simulink library "aerolibgravity2"  (Simulink 6.0)
settings: Solver=ode45  SolverMode=SingleTasking  StartTime=0.0  StopTime=10.0  RelTol=1e-3
values from neighbouring files (symbols this model uses):
  s = aeroliblist    [asbhelp.m]
undefined symbols (not defined in the file or in its folder): aeroassertmsg, c, cd, epoch, fm, fn, k, m, maxdef, snorm
libraries: simulink x9, aerolibconvert x8, aerolibutil x2
(part 1 of 2)
settings Model: Creator=sgage  LastModifiedBy=sgage  ExtModeAutoUpdateStatusClock=off  ProdHWDeviceType=Specified
settings DataIOCC: SignalLoggingName=logsOut
settings OptimizationCC: BooleanDataType=off
settings DebuggingCC: CheckExecutionContextPreStartOutputMsg=on  CheckExecutionContextRuntimeOutputMsg=on  SolverPrmCheckMsg=none
settings HardwareCC: ProdHWDeviceType=Specified  TargetUnknown=on
settings GRTTargetCC: LifeSpan=inf
settings SFSimCC: SFSimApplyToAllLibs=on  SFSimBuildMode=Incremental

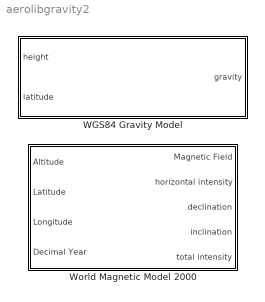
== system aerolibgravity2 ==
  WGS84 Gravity Model : Subsystem  PropExecContextAcrossSSBoundary=on  mask(WGS84 Gravity Model){model=WGS84 Taylor Series, units=Metric (MKS), no_atmos=on, precessing=on, month=February, day=1, year=2000, no_centrifugal=on, action=Warning}
      mask prompts: model "Type of gravity model:"; no_atmos "Exclude Earth's atmosphere"; precessing "Precessing reference frame"; no_centrifugal "No centrifugal effects"; action "Action for out of range input:"
      mask help:
      | Calculate Earth's gravity at a specific location using World Geodetic System (WGS 84).
      |
      | The WGS 84 model is defined as a geocentric equipotential ellipsoid. This model can be found in NIMA TR8350.2,  "Department of Defense World Geodetic System 1984, Its Definition and Relationship with Local Geodetic Systems."
      |
      | Height is entered in the same unit system as selected for gravity. Latitude and longitude (if required) are entered in degrees.
      mask init:
      | [str,ports] = aeroicon('aeroblkgravity','icon');
      mask Help: web(asbhelp);
      mask StyleString: popup(WGS84 Taylor Series|WGS84 Close Approximation|WGS84 Exact),popup(Metric (MKS)|English),checkbox,checkbox,popup(January|February|March|April|May|June|July|August|September|October|November|December),edit,edit,checkbox,popup(None|Warning|Error)
      mask CallbackString: aeroicon('aeroblkgravity')|||aeroicon('aeroblkgravity')|aeroicon('aeroblkgravity')|aeroicon('aeroblkgravity')|aeroicon('aeroblkgravity')||
      mask Display:
      | disp(str);
      | port_label(ports(1).type,ports(1).port,ports(1).txt,'texmode','on');
      | port_label(ports(2).type,ports(2).port,ports(2).txt,'texmode','on');
      | port_label(ports(3).type,ports(3).port,ports(3).txt,'texmode','on');
      | port_label(ports(4).type,ports(4).port,ports(4).txt,'texmode','on');
  World Magnetic Model 2000 : Subsystem  PropExecContextAcrossSSBoundary=on  mask(World Magnetic Model 2000){units=Metric (MKS), time_in=on, month=January, day=1, year=2000, action=Error, h_out=on, dec_out=on, inc_out=on, ti_out=on}
      mask prompts: time_in "Input decimal year"; action "Action for out of range input:"; h_out "Output horizontal intensity"; dec_out "Output declination"; inc_out "Output inclination"; ti_out "Output total intensity"
      mask help:
      | Calculate the Earth's magnetic field at a specific location and time using the World Magnetic Model (WMM). This model is valid for the year 2000 through the year 2005.
      |
      | The WMM-2000 can be found on the web at http://wmm.ngdc.noaa.gov/DoDWMM.shtml and in "British Geological Survey, Technical Report WM/00/17R, Geomagnetism Series".
      |
      | Height is entered in length units of selected unit system. Latitude and longitude are entered in degrees.
      mask init:
      | [ports,dyear,maxdef,epoch,c,cd,fn,fm,snorm,k]=aeroicon('aeroblkwmm','icon');
      mask Help: web(asbhelp);
      mask StyleString: popup(Metric (MKS)|English),checkbox,popup(January|February|March|April|May|June|July|August|September|October|November|December),popup(1|2|3|4|5|6|7|8|9|10|11|12|13|14|15|16|17|18|19|20|21|22|23|24|25|26|27|28|29|30|31),popup(2000|2001|2002|2003|2004|2005),popup(None|Warning|Error),checkbox,checkbox,checkbox,checkbox
      mask CallbackString: |aeroicon('aeroblkwmm');|aeroicon('aeroblkwmm');|aeroicon('aeroblkwmm');|aeroicon('aeroblkwmm');|||||
      mask Display:
      | port_label(ports(1).type,ports(1).port,ports(1).txt);
      | port_label(ports(2).type,ports(2).port,ports(2).txt);
      | port_label(ports(3).type,ports(3).port,ports(3).txt);
      | port_label(ports(4).type,ports(4).port,ports(4).txt);
      | port_label(ports(5).type,ports(5).port,ports(5).txt);
      | port_label(ports(6).type,ports(6).port,ports(6).txt);
      | port_label(ports(7).type,ports(7).port,ports(7).txt);
      | port_label(ports(8).type,ports(8).port,ports(8).txt);
      | port_label(ports(9).type,ports(9).port,ports(9).txt);

== system aerolibgravity2/WGS84 Gravity Model ==
  height : Inport  LatchInput=off
  latitude : Inport  Port=2  LatchInput=off
  Acceleration Conversion : aerolibconvert/Acceleration Conversion  IU=m/s^2  OU=m/s^2
  Angle Conversion : aerolibconvert/Angle Conversion  IU=deg  OU=rad
  Angle Conversion1 : aerolibconvert/Angle Conversion  IU=deg  OU=rad
  Length Conversion : aerolibconvert/Length Conversion  IU=m  OU=m
  WGS84 Gravity S-Function : S-Function  FunctionName=saerogravity2  Parameters=model,units,no_atmos,precessing,month,day,year,no_centrifugal,action  SFunctionModules=aerogravitywgs84
  longitude : Ground
  gravity : Outport
  wires:
  WGS84 Gravity S-Function/1 -> Acceleration Conversion/1
  height/1 -> Length Conversion/1
  latitude/1 -> Angle Conversion1/1
  Length Conversion/1 -> WGS84 Gravity S-Function/1
  Acceleration Conversion/1 -> gravity/1
  Angle Conversion1/1 -> WGS84 Gravity S-Function/2
  longitude/1 -> Angle Conversion/1
  Angle Conversion/1 -> WGS84 Gravity S-Function/3

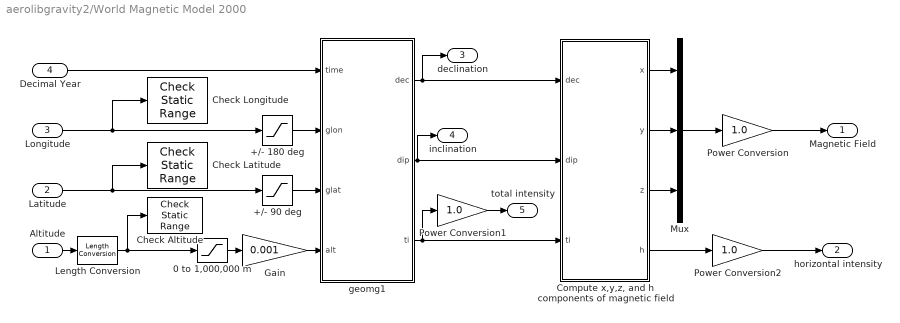
== system aerolibgravity2/World Magnetic Model 2000 ==
  Altitude : Inport  LatchInput=off
  Latitude : Inport  Port=2  LatchInput=off
  Longitude : Inport  Port=3  LatchInput=off
  Decimal Year : Inport  Port=4  LatchInput=off
  +/- 180 deg : Saturate  UpperLimit=180.0  LowerLimit=-180.0
  +/- 90 deg : Saturate  UpperLimit=90.0  LowerLimit=-90.0
  0 to 1,000,000 m : Saturate  UpperLimit=1000000.0  LowerLimit=0
  Check Altitude : simulink/Model Verification/Check  Static Range  Description=0 <= u <= 1000000  max=1000000  max_included=on  min=0  min_included=on  enabled=on  callback=aeroassertmsg('aeroblkwmm','alt');  stopWhenAssertionFail=on  export=off  icon=graphic
  Check Latitude : simulink/Model Verification/Check  Static Range  Description=-90 <= u <= 90  max=90  max_included=on  min=-90  min_included=on  enabled=on  callback=aeroassertmsg('aeroblkwmm','lat');  stopWhenAssertionFail=on  export=off  icon=graphic
  Check Longitude : simulink/Model Verification/Check  Static Range  Description=-180 <= u <= 180  max=180  max_included=on  min=-180  min_included=on  enabled=on  callback=aeroassertmsg('aeroblkwmm','lon');  stopWhenAssertionFail=on  export=off  icon=graphic
  "Compute x,y,z, and h components of magnetic field" : Subsystem  PropExecContextAcrossSSBoundary=on
  Gain : Gain  Gain=0.001  SaturateOnIntegerOverflow=on
  Length Conversion : aerolibconvert/Length Conversion  IU=m  OU=m
  Mux : Mux  Inputs=3
  Power Conversion : Gain  Gain=1.0  SaturateOnIntegerOverflow=on
  Power Conversion1 : Gain  Gain=1.0  SaturateOnIntegerOverflow=on
  Power Conversion2 : Gain  Gain=1.0  SaturateOnIntegerOverflow=on
  geomg1 : Subsystem  PropExecContextAcrossSSBoundary=on
  Magnetic Field : Outport
  horizontal intensity : Outport  Port=2
  declination : Outport  Port=3
  inclination : Outport  Port=4
  total intensity : Outport  Port=5
  wires:
  0 to 1,000,000 m/1 -> Gain/1
  +/- 180 deg/1 -> geomg1/2(glon)
  +/- 90 deg/1 -> geomg1/3(glat)
  Power Conversion2/1 -> horizontal intensity/1
  Power Conversion1/1 -> total intensity/1
  Power Conversion/1 -> Magnetic Field/1
  Mux/1 -> Power Conversion/1
  geomg1/1(dec) -> declination/1, "Compute x,y,z, and h components of magnetic field"/1(dec)
  Gain/1 -> geomg1/4(alt)
  Longitude/1 -> Check Longitude/1, +/- 180 deg/1
  Latitude/1 -> Check Latitude/1, +/- 90 deg/1
  geomg1/3(ti) -> Power Conversion1/1, "Compute x,y,z, and h components of magnetic field"/3(ti)
  geomg1/2(dip) -> inclination/1, "Compute x,y,z, and h components of magnetic field"/2(dip)
  Decimal Year/1 -> geomg1/1(time)
  "Compute x,y,z, and h components of magnetic field"/4(h) -> Power Conversion2/1
  "Compute x,y,z, and h components of magnetic field"/3(z) -> Mux/3
  "Compute x,y,z, and h components of magnetic field"/2(y) -> Mux/2
  "Compute x,y,z, and h components of magnetic field"/1(x) -> Mux/1
  Length Conversion/1 -> Check Altitude/1, 0 to 1,000,000 m/1
  Altitude/1 -> Length Conversion/1

== system aerolibgravity2/World Magnetic Model 2000/Compute x,y,z, and h components of magnetic field ==
  dec : Inport  LatchInput=off
  dip : Inport  Port=2  LatchInput=off
  ti : Inport  Port=3  LatchInput=off
  Demux : Demux  Outputs=2
  Demux1 : Demux  Outputs=2
  Mux : Mux  Inputs=2
  SinCos : aerolibutil/SinCos
  h1 : Product  SaturateOnIntegerOverflow=on
  rTd : Gain  Gain=0.017453292  SaturateOnIntegerOverflow=on
  x1 : Product  SaturateOnIntegerOverflow=on
  y1 : Product  SaturateOnIntegerOverflow=on
  z1 : Product  SaturateOnIntegerOverflow=on
  x : Outport
  y : Outport  Port=2
  z : Outport  Port=3
  h : Outport  Port=4
  wires:
  z1/1 -> z/1
  x1/1 -> x/1
  dip/1 -> Mux/2
  y1/1 -> y/1
  dec/1 -> Mux/1
  Demux1/1 -> y1/1
  Demux1/2 -> z1/1
  Demux/1 -> x1/1
  h1/1 -> h/1, x1/2, y1/2
  Demux/2 -> h1/1
  ti/1 -> h1/2, z1/2
  SinCos/2 -> Demux/1
  SinCos/1 -> Demux1/1
  rTd/1 -> SinCos/1
  Mux/1 -> rTd/1

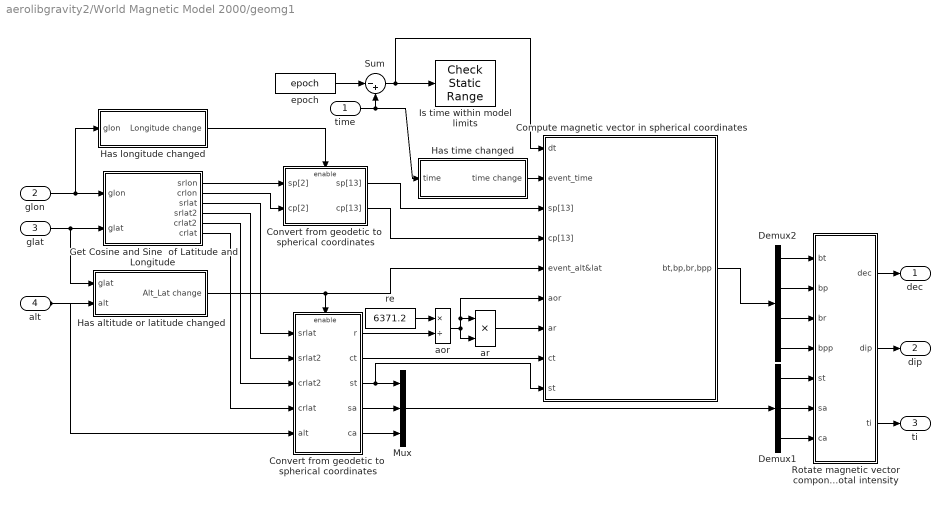
== system aerolibgravity2/World Magnetic Model 2000/geomg1 ==
  time : Inport  LatchInput=off
  glon : Inport  Port=2  LatchInput=off
  glat : Inport  Port=3  LatchInput=off
  alt : Inport  Port=4  LatchInput=off
  Compute magnetic vector in spherical coordinates : Subsystem  TreatAsAtomicUnit=on  PropExecContextAcrossSSBoundary=on
  Convert from geodetic to  spherical coordinates : Subsystem  TreatAsAtomicUnit=on  PropExecContextAcrossSSBoundary=on
  "Convert from geodetic to  spherical coordinates " : Subsystem  PropExecContextAcrossSSBoundary=on
  Demux1 : Demux  Outputs=3
  Demux2 : Demux
  Get Cosine and Sine  of Latitude and Longitude : Subsystem  PropExecContextAcrossSSBoundary=on
  Has altitude or latitude changed : Subsystem  PropExecContextAcrossSSBoundary=on
  "Has longitude changed " : Subsystem  PropExecContextAcrossSSBoundary=on
  Has time changed : Subsystem  AncestorBlock="aerolibatmosratios/WMM 2000/geomg1_/Determine Whether To  Convert Coordinates"  PropExecContextAcrossSSBoundary=on
  Is time within model limits : simulink/Model Verification/Check  Static Range  Description=0 <= u <= 5  max=5  max_included=on  min=0  min_included=on  enabled=on  callback=aeroassertmsg('aeroblkwmm','time');  stopWhenAssertionFail=on  export=off  icon=graphic
  Mux : Mux  Inputs=3
  "Rotate magnetic vector components  to geodetic from spherical and  compute declination, inclination  and total intensity" : Subsystem  PropExecContextAcrossSSBoundary=on
  Sum : Sum  Inputs=|-+  SaturateOnIntegerOverflow=on
  aor : Product  Inputs=*/  SaturateOnIntegerOverflow=on
  ar : Product  SaturateOnIntegerOverflow=on
  epoch : Constant  Value=epoch
  re : Constant  Value=6371.2
  dec : Outport
  dip : Outport  Port=2
  ti : Outport  Port=3
  wires:
  Demux2/3 -> "Rotate magnetic vector components  to geodetic from spherical and  compute declination, inclination  and total intensity"/3(br)
  Demux2/2 -> "Rotate magnetic vector components  to geodetic from spherical and  compute declination, inclination  and total intensity"/2(bp)
  Compute magnetic vector in spherical coordinates/1(bt,bp,br,bpp) -> Demux2/1
  Demux1/3 -> "Rotate magnetic vector components  to geodetic from spherical and  compute declination, inclination  and total intensity"/7(ca)
  Demux1/2 -> "Rotate magnetic vector components  to geodetic from spherical and  compute declination, inclination  and total intensity"/6(sa)
  Demux1/1 -> "Rotate magnetic vector components  to geodetic from spherical and  compute declination, inclination  and total intensity"/5(st)
  Demux2/4 -> "Rotate magnetic vector components  to geodetic from spherical and  compute declination, inclination  and total intensity"/4(bpp)
  Demux2/1 -> "Rotate magnetic vector components  to geodetic from spherical and  compute declination, inclination  and total intensity"/1(bt)
  Mux/1 -> Demux1/1
  Convert from geodetic to  spherical coordinates/5(ca) -> Mux/3
  Convert from geodetic to  spherical coordinates/4(sa) -> Mux/2
  Convert from geodetic to  spherical coordinates/3(st) -> Compute magnetic vector in spherical coordinates/9(st), Mux/1
  epoch/1 -> Sum/1
  Convert from geodetic to  spherical coordinates/2(ct) -> Compute magnetic vector in spherical coordinates/8(ct)
  Get Cosine and Sine  of Latitude and Longitude/6(crlat) -> Convert from geodetic to  spherical coordinates/4(crlat)
  Get Cosine and Sine  of Latitude and Longitude/3(srlat) -> Convert from geodetic to  spherical coordinates/1(srlat)
  "Rotate magnetic vector components  to geodetic from spherical and  compute declination, inclination  and total intensity"/3(ti) -> ti/1
  "Rotate magnetic vector components  to geodetic from spherical and  compute declination, inclination  and total intensity"/2(dip) -> dip/1
  "Rotate magnetic vector components  to geodetic from spherical and  compute declination, inclination  and total intensity"/1(dec) -> dec/1
  ar/1 -> Compute magnetic vector in spherical coordinates/7(ar)
  re/1 -> aor/1
  Convert from geodetic to  spherical coordinates/1(r) -> aor/2
  aor/1 -> ar/1, Compute magnetic vector in spherical coordinates/6(aor), ar/2
  "Convert from geodetic to  spherical coordinates "/2(cp[13]) -> Compute magnetic vector in spherical coordinates/4(cp[13])
  "Convert from geodetic to  spherical coordinates "/1(sp[13]) -> Compute magnetic vector in spherical coordinates/3(sp[13])
  Has altitude or latitude changed/1(Alt_Lat change) -> Compute magnetic vector in spherical coordinates/5(event_alt&lat), Convert from geodetic to  spherical coordinates/Enable
  Get Cosine and Sine  of Latitude and Longitude/5(crlat2) -> Convert from geodetic to  spherical coordinates/3(crlat2)
  Get Cosine and Sine  of Latitude and Longitude/4(srlat2) -> Convert from geodetic to  spherical coordinates/2(srlat2)
  Get Cosine and Sine  of Latitude and Longitude/2(crlon) -> "Convert from geodetic to  spherical coordinates "/2(cp[2])
  Get Cosine and Sine  of Latitude and Longitude/1(srlon) -> "Convert from geodetic to  spherical coordinates "/1(sp[2])
  alt/1 -> Convert from geodetic to  spherical coordinates/5(alt), Has altitude or latitude changed/2(alt)
  glat/1 -> Get Cosine and Sine  of Latitude and Longitude/2(glat), Has altitude or latitude changed/1(glat)
  glon/1 -> Get Cosine and Sine  of Latitude and Longitude/1(glon), "Has longitude changed "/1(glon)
  "Has longitude changed "/1(Longitude change) -> "Convert from geodetic to  spherical coordinates "/Enable
  Has time changed/1(time change) -> Compute magnetic vector in spherical coordinates/2(event_time)
  time/1 -> Sum/2, Has time changed/1(time)
  Sum/1 -> Compute magnetic vector in spherical coordinates/1(dt), Is time within model limits/1

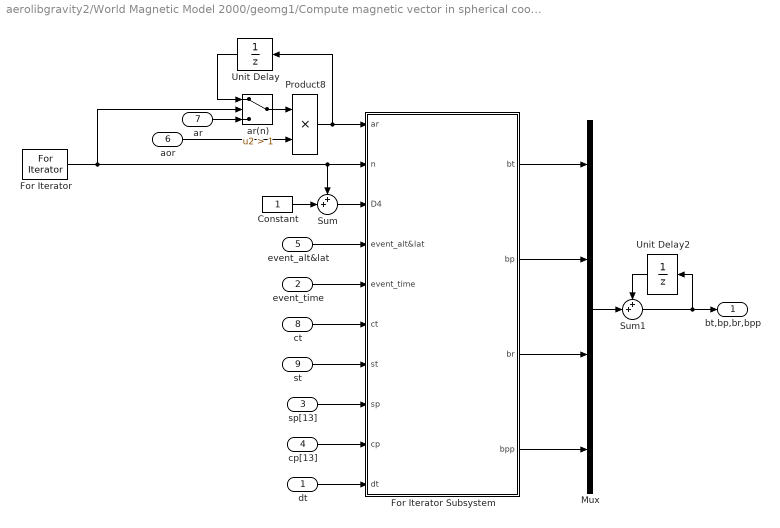
== system aerolibgravity2/World Magnetic Model 2000/geomg1/Compute magnetic vector in spherical coordinates ==
  dt : Inport  LatchInput=off
  event_time : Inport  Port=2  LatchInput=off
  sp[13] : Inport  Port=3  LatchInput=off
  cp[13] : Inport  Port=4  LatchInput=off
  event_alt&lat : Inport  Port=5  LatchInput=off
  aor : Inport  Port=6  LatchInput=off
  ar : Inport  Port=7  LatchInput=off
  ct : Inport  Port=8  LatchInput=off
  st : Inport  Port=9  LatchInput=off
  Constant : Constant
  For Iterator : ForIterator  ResetStates=reset  IterationLimit=maxdef
  For Iterator Subsystem : Subsystem  TreatAsAtomicUnit=on  PropExecContextAcrossSSBoundary=on
  Mux : Mux
  Product8 : Product  SaturateOnIntegerOverflow=on
  Sum : Sum  Inputs=++|  SaturateOnIntegerOverflow=on
  Sum1 : Sum  Inputs=++|  SaturateOnIntegerOverflow=on
  Unit Delay : UnitDelay  Orientation=left  SampleTime=-1
  Unit Delay2 : UnitDelay  Orientation=left  X0=[0 0 0 0]  SampleTime=-1
  ar(n) : Switch  Criteria=u2 > Threshold  Threshold=1  SaturateOnIntegerOverflow=on
  bt,bp,br,bpp : Outport
  wires:
  Sum1/1 -> Unit Delay2/1, bt,bp,br,bpp/1
  Unit Delay2/1 -> Sum1/1
  Mux/1 -> Sum1/2
  For Iterator Subsystem/4(bpp) -> Mux/4
  For Iterator Subsystem/3(br) -> Mux/3
  For Iterator Subsystem/2(bp) -> Mux/2
  For Iterator Subsystem/1(bt) -> Mux/1
  dt/1 -> For Iterator Subsystem/10(dt)
  cp[13]/1 -> For Iterator Subsystem/9(cp)
  sp[13]/1 -> For Iterator Subsystem/8(sp)
  st/1 -> For Iterator Subsystem/7(st)
  ct/1 -> For Iterator Subsystem/6(ct)
  Constant/1 -> Sum/2
  Sum/1 -> For Iterator Subsystem/3(D4)
  ar(n)/1 -> Product8/1
  Product8/1 -> For Iterator Subsystem/1(ar), Unit Delay/1
  Unit Delay/1 -> ar(n)/1
  aor/1 -> Product8/2
  event_time/1 -> For Iterator Subsystem/5(event_time)
  ar/1 -> ar(n)/3
  event_alt&lat/1 -> For Iterator Subsystem/4(event_alt&lat)
  For Iterator/1 -> Sum/1, For Iterator Subsystem/2(n), ar(n)/2

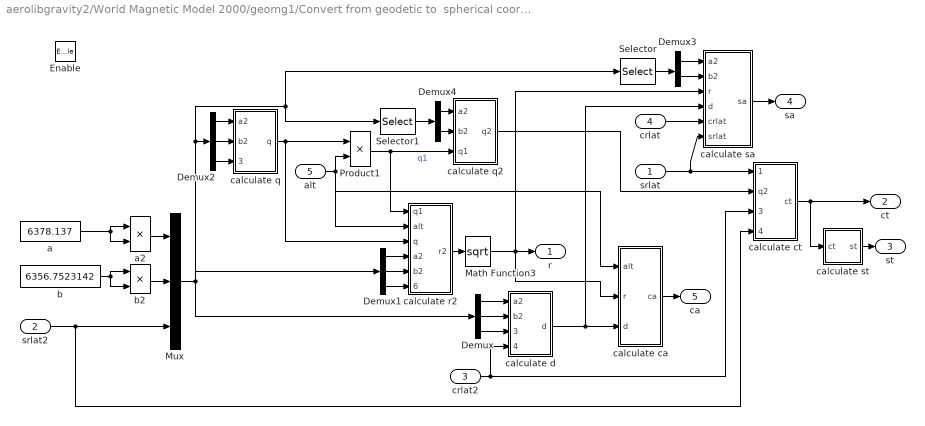
== system aerolibgravity2/World Magnetic Model 2000/geomg1/Convert from geodetic to  spherical coordinates ==
  srlat : Inport  LatchInput=off
  srlat2 : Inport  Port=2  LatchInput=off
  crlat2 : Inport  Port=3  LatchInput=off
  crlat : Inport  Port=4  LatchInput=off
  alt : Inport  Port=5  LatchInput=off
  Enable : EnablePort
  Demux : Demux  Outputs=3
  Demux1 : Demux  Outputs=3
  Demux2 : Demux  Outputs=3
  Demux3 : Demux  Outputs=2
  Demux4 : Demux  Outputs=2
  Math Function3 : Math  Operator=sqrt  SaturateOnIntegerOverflow=on
  Mux : Mux  Inputs=3
  Product1 : Product  SaturateOnIntegerOverflow=on
  Selector : Selector  Elements=[1 2]  InputPortWidth=3
  Selector1 : Selector  Elements=[1 2]  InputPortWidth=3
  a : Constant  Value=6378.137
  a2 : Product  SaturateOnIntegerOverflow=on
  b : Constant  Value=6356.7523142
  b2 : Product  SaturateOnIntegerOverflow=on
  calculate ca : Subsystem  PropExecContextAcrossSSBoundary=on
  calculate ct : Subsystem  PropExecContextAcrossSSBoundary=on
  calculate d : Subsystem  PropExecContextAcrossSSBoundary=on
  calculate q : Subsystem  PropExecContextAcrossSSBoundary=on
  calculate q2 : Subsystem  PropExecContextAcrossSSBoundary=on
  calculate r2 : Subsystem  PropExecContextAcrossSSBoundary=on
  calculate sa : Subsystem  PropExecContextAcrossSSBoundary=on
  calculate st : Subsystem  PropExecContextAcrossSSBoundary=on
  r : Outport
  ct : Outport  Port=2
  st : Outport  Port=3
  sa : Outport  Port=4
  ca : Outport  Port=5
  wires:
  Demux/3 -> calculate d/3(srlat2)
  Demux4/2 -> calculate q2/2(b2)
  Demux4/1 -> calculate q2/1(a2)
  Selector1/1 -> Demux4/1
  Selector/1 -> Demux3/1
  Demux3/2 -> calculate sa/2(b2)
  Demux3/1 -> calculate sa/1(a2)
  Mux/1 -> Selector/1, Selector1/1, Demux2/1, Demux/1, Demux1/1
  Demux2/3 -> calculate q/3(srlat2)
  Demux2/2 -> calculate q/2(b2)
  Demux2/1 -> calculate q/1(a2)
  Demux1/3 -> calculate r2/6(srlat2)
  Demux1/2 -> calculate r2/5(b2)
  Demux1/1 -> calculate r2/4(a2)
  Demux/1 -> calculate d/1(a2)
  Demux/2 -> calculate d/2(b2)
  calculate q2/1(q2) -> calculate ct/2(q2)
  b2/1 -> Mux/2
  b/1 -> b2/1, b2/2
  a2/1 -> Mux/1
  a/1 -> a2/1, a2/2
  calculate sa/1(sa) -> sa/1
  crlat/1 -> calculate sa/5(crlat)
  calculate ca/1(ca) -> ca/1
  calculate d/1(d) -> calculate sa/4(d), calculate ca/3(d)
  Math Function3/1 -> calculate ca/2(r), calculate sa/3(r), r/1
  calculate r2/1(r2) -> Math Function3/1
  calculate st/1(st) -> st/1
  calculate ct/1(ct) -> calculate st/1(ct), ct/1
  srlat/1 -> calculate sa/6(srlat), calculate ct/1(srlat)
  crlat2/1 -> calculate ct/3(crlat2), calculate d/4(crlat2)
  alt/1 -> calculate r2/2(alt), calculate ca/1(alt), Product1/2
  Product1/1 -> calculate r2/1(q1), calculate q2/3(q1)  "q1"
  calculate q/1(q) -> calculate r2/3(q), Product1/1
  srlat2/1 -> Mux/3, calculate ct/4(srlat2)

== system aerolibgravity2/World Magnetic Model 2000/geomg1/Convert from geodetic to  spherical coordinates  ==
  sp[2] : Inport  LatchInput=off
  cp[2] : Inport  Port=2  LatchInput=off
  Enable : EnablePort
  For Iterator Subsystem : Subsystem  AncestorBlock=aerolibatmosratios/WMM 2000/geomg1_/For Iterator Subsystem  TreatAsAtomicUnit=on  PropExecContextAcrossSSBoundary=on
  Mux : Mux  Inputs=3
  Mux1 : Mux  Inputs=3
  cp[1] : Constant
  sp[1] : Constant  Value=0
  sp[13] : Outport  InitialOutput=[ zeros(1,13) ]
  cp[13] : Outport  Port=2  InitialOutput=[ zeros(1,13) ]
  wires:
  sp[1]/1 -> Mux1/1
  cp[1]/1 -> Mux/1
  Mux/1 -> cp[13]/1
  For Iterator Subsystem/2(cp[11]) -> Mux/3
  For Iterator Subsystem/1(sp[11]) -> Mux1/3
  cp[2]/1 -> For Iterator Subsystem/2(cp[2]), Mux/2
  sp[2]/1 -> For Iterator Subsystem/1(sp[2]), Mux1/2
  Mux1/1 -> sp[13]/1

== system aerolibgravity2/World Magnetic Model 2000/geomg1/Get Cosine and Sine  of Latitude and Longitude ==
  glon : Inport  LatchInput=off
  glat : Inport  Port=2  LatchInput=off
  Angle Conversion : aerolibconvert/Angle Conversion  IU=deg  OU=rad
  Demux : Demux  Outputs=2
  Demux1 : Demux  Outputs=2
  Mux : Mux  Inputs=2
  Product : Product  SaturateOnIntegerOverflow=on
  Product1 : Product  SaturateOnIntegerOverflow=on
  SinCos : aerolibutil/SinCos
  srlon : Outport
  crlon : Outport  Port=2
  srlat : Outport  Port=3
  srlat2 : Outport  Port=4
  crlat2 : Outport  Port=5
  crlat : Outport  Port=6
  wires:
  Demux1/2 -> Product1/2, Product1/1, crlat/1
  Demux/2 -> Product/2, Product/1, srlat/1
  Product1/1 -> crlat2/1
  Product/1 -> srlat2/1
  Demux1/1 -> crlon/1
  Demux/1 -> srlon/1
  glat/1 -> Mux/2
  glon/1 -> Mux/1
  SinCos/2 -> Demux1/1
  SinCos/1 -> Demux/1
  Mux/1 -> Angle Conversion/1
  Angle Conversion/1 -> SinCos/1

== system aerolibgravity2/World Magnetic Model 2000/geomg1/Has altitude or latitude changed ==
  glat : Inport  LatchInput=off
  alt : Inport  Port=2  LatchInput=off
  Logical Operator : Logic  Operator=OR  AllPortsSameDT=off
  Relational Operator : RelationalOperator  Operator=~=
  Relational Operator1 : RelationalOperator  Operator=~=
  oalt : Memory  X0=-1000
  olat : Memory  X0=-1000
  Alt_Lat change : Outport
  wires:
  Logical Operator/1 -> Alt_Lat change/1
  glat/1 -> olat/1, Relational Operator/1
  Relational Operator1/1 -> Logical Operator/2
  Relational Operator/1 -> Logical Operator/1
  oalt/1 -> Relational Operator1/2
  olat/1 -> Relational Operator/2
  alt/1 -> oalt/1, Relational Operator1/1

== system aerolibgravity2/World Magnetic Model 2000/geomg1/Has longitude changed  ==
  glon : Inport  LatchInput=off
  Relational Operator : RelationalOperator  Operator=~=
  olon : Memory  X0=-1000
  Longitude change : Outport
  wires:
  Relational Operator/1 -> Longitude change/1
  glon/1 -> olon/1, Relational Operator/1
  olon/1 -> Relational Operator/2

== system aerolibgravity2/World Magnetic Model 2000/geomg1/Has time changed ==
  time : Inport  LatchInput=off
  Relational Operator : RelationalOperator  Operator=~=
  otime : Memory  X0=-1000
  time change : Outport
  wires:
  otime/1 -> Relational Operator/2
  time/1 -> Relational Operator/1, otime/1
  Relational Operator/1 -> time change/1

== system aerolibgravity2/World Magnetic Model 2000/geomg1/Rotate magnetic vector components  to geodetic from spherical and  compute declination, inclination  and total intensity ==
  bt : Inport  LatchInput=off
  bp : Inport  Port=2  LatchInput=off
  br : Inport  Port=3  LatchInput=off
  bpp : Inport  Port=4  LatchInput=off
  st : Inport  Port=5  LatchInput=off
  sa : Inport  Port=6  LatchInput=off
  ca : Inport  Port=7  LatchInput=off
  Calculate bx : Subsystem  PropExecContextAcrossSSBoundary=on
  Calculate by : Subsystem  PropExecContextAcrossSSBoundary=on
  Calculate bz : Subsystem  AncestorBlock=aerolibatmosratios/WMM 2000/geomg1_/Subsystem1/Calculate bx  PropExecContextAcrossSSBoundary=on
  "Compute declination, inclination,  and total intensity" : Subsystem  PropExecContextAcrossSSBoundary=on
  Demux : Demux
  Demux1 : Demux
  Mux : Mux
  dec : Outport
  dip : Outport  Port=2
  ti : Outport  Port=3
  wires:
  "Compute declination, inclination,  and total intensity"/2(dip) -> dip/1
  "Compute declination, inclination,  and total intensity"/1(dec) -> dec/1
  Calculate bz/1(bz) -> "Compute declination, inclination,  and total intensity"/3(bz)
  Calculate bx/1(bx) -> "Compute declination, inclination,  and total intensity"/2(bx)
  Calculate by/1(by) -> "Compute declination, inclination,  and total intensity"/1(by)
  "Compute declination, inclination,  and total intensity"/3(ti) -> ti/1
  Demux1/4 -> Calculate bz/4(br)
  Demux1/3 -> Calculate bz/3(bt)
  Demux1/2 -> Calculate bz/2(sa)
  Demux1/1 -> Calculate bz/1(ca)
  Mux/1 -> Demux1/1, Demux/1
  Demux/4 -> Calculate bx/4(br)
  Demux/3 -> Calculate bx/3(bt)
  Demux/2 -> Calculate bx/2(sa)
  Demux/1 -> Calculate bx/1(ca)
  br/1 -> Mux/4
  bt/1 -> Mux/3
  sa/1 -> Mux/2
  ca/1 -> Mux/1
  bp/1 -> Calculate by/1(bp)
  bpp/1 -> Calculate by/3(bpp)
  st/1 -> Calculate by/2(st)

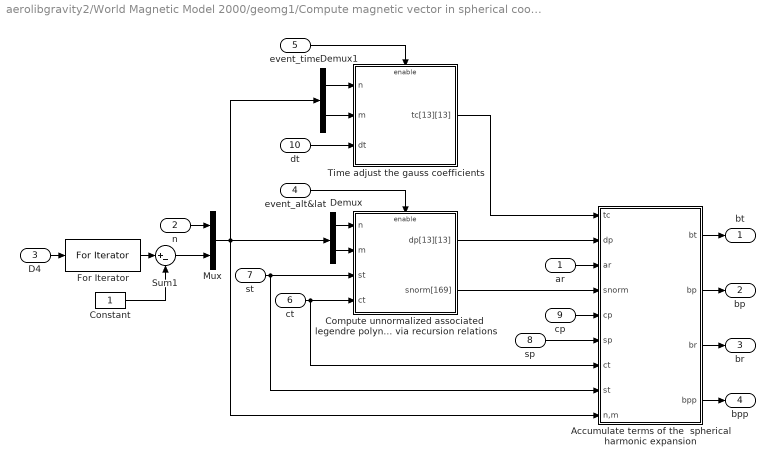
== system aerolibgravity2/World Magnetic Model 2000/geomg1/Compute magnetic vector in spherical coordinates/For Iterator Subsystem ==
  ar : Inport  LatchInput=off
  n : Inport  Port=2  LatchInput=off
  D4 : Inport  Port=3  LatchInput=off
  event_alt&lat : Inport  Port=4  LatchInput=off
  event_time : Inport  Port=5  LatchInput=off
  ct : Inport  Port=6  LatchInput=off
  st : Inport  Port=7  LatchInput=off
  sp : Inport  Port=8  LatchInput=off
  cp : Inport  Port=9  LatchInput=off
  dt : Inport  Port=10  LatchInput=off
  Accumulate terms of the  spherical harmonic expansion : Subsystem  PropExecContextAcrossSSBoundary=on
  Compute unnormalized associated  legendre polynomials and  derivatives via recursion relations : Subsystem  TreatAsAtomicUnit=on  PropExecContextAcrossSSBoundary=on
  Constant : Constant
  Demux : Demux  Outputs=2
  Demux1 : Demux  Outputs=2
  For Iterator : ForIterator  ResetStates=reset  IterationSource=external  IterationLimit=maxdef
  Mux : Mux  Inputs=2
  Sum1 : Sum  Inputs=|+-  SaturateOnIntegerOverflow=on
  Time adjust the gauss coefficients : Subsystem  TreatAsAtomicUnit=on  PropExecContextAcrossSSBoundary=on
  bt : Outport
  bp : Outport  Port=2
  br : Outport  Port=3
  bpp : Outport  Port=4
  wires:
  Accumulate terms of the  spherical harmonic expansion/4(bpp) -> bpp/1
  Sum1/1 -> Mux/2
  For Iterator/1 -> Sum1/1
  Demux1/2 -> Time adjust the gauss coefficients/2(m)
  Demux1/1 -> Time adjust the gauss coefficients/1(n)
  Demux/2 -> Compute unnormalized associated  legendre polynomials and  derivatives via recursion relations/2(m)
  Demux/1 -> Compute unnormalized associated  legendre polynomials and  derivatives via recursion relations/1(n)
  n/1 -> Mux/1
  Mux/1 -> Accumulate terms of the  spherical harmonic expansion/9(n,m), Demux1/1, Demux/1
  Time adjust the gauss coefficients/1(tc[13][13]) -> Accumulate terms of the  spherical harmonic expansion/1(tc)
  ar/1 -> Accumulate terms of the  spherical harmonic expansion/3(ar)
  Accumulate terms of the  spherical harmonic expansion/2(bp) -> bp/1
  Accumulate terms of the  spherical harmonic expansion/1(bt) -> bt/1
  Accumulate terms of the  spherical harmonic expansion/3(br) -> br/1
  Compute unnormalized associated  legendre polynomials and  derivatives via recursion relations/1(dp[13][13]) -> Accumulate terms of the  spherical harmonic expansion/2(dp)
  Compute unnormalized associated  legendre polynomials and  derivatives via recursion relations/2(snorm[169]) -> Accumulate terms of the  spherical harmonic expansion/4(snorm)
  sp/1 -> Accumulate terms of the  spherical harmonic expansion/6(sp)
  cp/1 -> Accumulate terms of the  spherical harmonic expansion/5(cp)
  ct/1 -> Accumulate terms of the  spherical harmonic expansion/7(ct), Compute unnormalized associated  legendre polynomials and  derivatives via recursion relations/4(ct)
  st/1 -> Accumulate terms of the  spherical harmonic expansion/8(st), Compute unnormalized associated  legendre polynomials and  derivatives via recursion relations/3(st)
  dt/1 -> Time adjust the gauss coefficients/3(dt)
  event_time/1 -> Time adjust the gauss coefficients/Enable
  Constant/1 -> Sum1/2
  event_alt&lat/1 -> Compute unnormalized associated  legendre polynomials and  derivatives via recursion relations/Enable
  D4/1 -> For Iterator/1

== system aerolibgravity2/World Magnetic Model 2000/geomg1/Convert from geodetic to  spherical coordinates/calculate ca ==
  alt : Inport  LatchInput=off
  r : Inport  Port=2  LatchInput=off
  d : Inport  Port=3  LatchInput=off
  Product11 : Product  Inputs=/*  SaturateOnIntegerOverflow=on
  Sum8 : Sum  Inputs=|++  SaturateOnIntegerOverflow=on
  ca : Outport
  wires:
  Product11/1 -> ca/1
  d/1 -> Sum8/2
  alt/1 -> Sum8/1
  r/1 -> Product11/1
  Sum8/1 -> Product11/2

== system aerolibgravity2/World Magnetic Model 2000/geomg1/Convert from geodetic to  spherical coordinates/calculate ct ==
  srlat : Inport  LatchInput=off
  q2 : Inport  Port=2  LatchInput=off
  crlat2 : Inport  Port=3  LatchInput=off
  srlat2 : Inport  Port=4  LatchInput=off
  Math Function1 : Math  Operator=sqrt  SaturateOnIntegerOverflow=on
  Product3 : Product  SaturateOnIntegerOverflow=on
  Product4 : Product  Inputs=*/  SaturateOnIntegerOverflow=on
  Sum3 : Sum  Inputs=|++  SaturateOnIntegerOverflow=on
  ct : Outport
  wires:
  Product3/1 -> Sum3/2
  srlat2/1 -> Sum3/1
  q2/1 -> Product3/2
  crlat2/1 -> Product3/1
  Product4/1 -> ct/1
  srlat/1 -> Product4/1
  Math Function1/1 -> Product4/2
  Sum3/1 -> Math Function1/1

== system aerolibgravity2/World Magnetic Model 2000/geomg1/Convert from geodetic to  spherical coordinates/calculate d ==
  a2 : Inport  LatchInput=off
  b2 : Inport  Port=2  LatchInput=off
  srlat2 : Inport  Port=3  LatchInput=off
  crlat2 : Inport  Port=4  LatchInput=off
  Math Function4 : Math  Operator=sqrt  SaturateOnIntegerOverflow=on
  Product10 : Product  SaturateOnIntegerOverflow=on
  Product9 : Product  SaturateOnIntegerOverflow=on
  Sum7 : Sum  Inputs=++|  SaturateOnIntegerOverflow=on
  d : Outport
  wires:
  Math Function4/1 -> d/1  "d"
  srlat2/1 -> Product10/2
  b2/1 -> Product10/1
  a2/1 -> Product9/2
  crlat2/1 -> Product9/1
  Product10/1 -> Sum7/2
  Product9/1 -> Sum7/1
  Sum7/1 -> Math Function4/1

== system aerolibgravity2/World Magnetic Model 2000/geomg1/Convert from geodetic to  spherical coordinates/calculate q ==
  a2 : Inport  LatchInput=off
  b2 : Inport  Port=2  LatchInput=off
  srlat2 : Inport  Port=3  LatchInput=off
  Math Function : Math  Operator=sqrt  SaturateOnIntegerOverflow=on
  Product : Product  SaturateOnIntegerOverflow=on
  Sum : Sum  Inputs=|-+  SaturateOnIntegerOverflow=on
  Sum1 : Sum  Inputs=|-+  SaturateOnIntegerOverflow=on
  q : Outport
  wires:
  b2/1 -> Sum1/1
  Math Function/1 -> q/1  "q"
  a2/1 -> Sum1/2, Sum/2
  Sum1/1 -> Product/2  "c2"
  srlat2/1 -> Product/1
  Sum/1 -> Math Function/1
  Product/1 -> Sum/1

== system aerolibgravity2/World Magnetic Model 2000/geomg1/Convert from geodetic to  spherical coordinates/calculate q2 ==
  a2 : Inport  LatchInput=off
  b2 : Inport  Port=2  LatchInput=off
  q1 : Inport  Port=3  LatchInput=off
  Product2 : Product  Inputs=**//  SaturateOnIntegerOverflow=on
  Sum1 : Sum  Inputs=++|  SaturateOnIntegerOverflow=on
  Sum2 : Sum  Inputs=++|  SaturateOnIntegerOverflow=on
  q2 : Outport
  wires:
  Product2/1 -> q2/1  "q2"
  b2/1 -> Sum1/2
  q1/1 -> Sum1/1, Sum2/2
  a2/1 -> Sum2/1
  Sum2/1 -> Product2/2, Product2/1
  Sum1/1 -> Product2/3, Product2/4

== system aerolibgravity2/World Magnetic Model 2000/geomg1/Convert from geodetic to  spherical coordinates/calculate r2 ==
  q1 : Inport  Orientation=down  LatchInput=off
  alt : Inport  Port=2  LatchInput=off
  q : Inport  Port=3  LatchInput=off
  a2 : Inport  Port=4  LatchInput=off
  b2 : Inport  Port=5  LatchInput=off
  srlat2 : Inport  Orientation=up  Port=6  LatchInput=off
  Gain : Gain  Orientation=down  Gain=2  SaturateOnIntegerOverflow=on
  Product6 : Product  SaturateOnIntegerOverflow=on
  Product7 : Product  Inputs=//*  SaturateOnIntegerOverflow=on
  Product8 : Product  Orientation=up  SaturateOnIntegerOverflow=on
  Sum5 : Sum  Inputs=+++  SaturateOnIntegerOverflow=on
  Sum6 : Sum  Inputs=|+-  SaturateOnIntegerOverflow=on
  Sum9 : Sum  Inputs=|+-  SaturateOnIntegerOverflow=on
  a4 : Product  SaturateOnIntegerOverflow=on
  b4 : Product  SaturateOnIntegerOverflow=on
  r2 : Outport
  wires:
  b2/1 -> b4/1, b4/2
  b4/1 -> Sum9/2
  Sum5/1 -> r2/1  "r2"
  srlat2/1 -> Product8/2
  a2/1 -> a4/2, a4/1
  alt/1 -> Product6/1, Product6/2
  q/1 -> Product7/1, Product7/2
  q1/1 -> Gain/1
  a4/1 -> Sum6/1, Sum9/1
  Sum9/1 -> Product8/1  "c4"
  Product8/1 -> Sum6/2
  Sum6/1 -> Product7/3
  Product7/1 -> Sum5/3
  Gain/1 -> Sum5/1
  Product6/1 -> Sum5/2

== system aerolibgravity2/World Magnetic Model 2000/geomg1/Convert from geodetic to  spherical coordinates/calculate sa ==
  a2 : Inport  LatchInput=off
  b2 : Inport  Port=2  LatchInput=off
  r : Inport  Port=3  LatchInput=off
  d : Inport  Port=4  LatchInput=off
  crlat : Inport  Port=5  LatchInput=off
  srlat : Inport  Port=6  LatchInput=off
  Product12 : Product  Inputs=*//**  SaturateOnIntegerOverflow=on
  Sum1 : Sum  Inputs=|-+  SaturateOnIntegerOverflow=on
  sa : Outport
  wires:
  crlat/1 -> Product12/4
  Product12/1 -> sa/1
  a2/1 -> Sum1/2
  b2/1 -> Sum1/1
  srlat/1 -> Product12/5
  d/1 -> Product12/3
  r/1 -> Product12/2
  Sum1/1 -> Product12/1  "c2"

== system aerolibgravity2/World Magnetic Model 2000/geomg1/Convert from geodetic to  spherical coordinates/calculate st ==
  ct : Inport  LatchInput=off
  Constant : Constant
  Math Function2 : Math  Operator=sqrt  SaturateOnIntegerOverflow=on
  Product5 : Product  SaturateOnIntegerOverflow=on
  Sum4 : Sum  Inputs=|-+  SaturateOnIntegerOverflow=on
  st : Outport
  wires:
  Math Function2/1 -> st/1
  ct/1 -> Product5/2, Product5/1
  Constant/1 -> Sum4/2
  Sum4/1 -> Math Function2/1
  Product5/1 -> Sum4/1

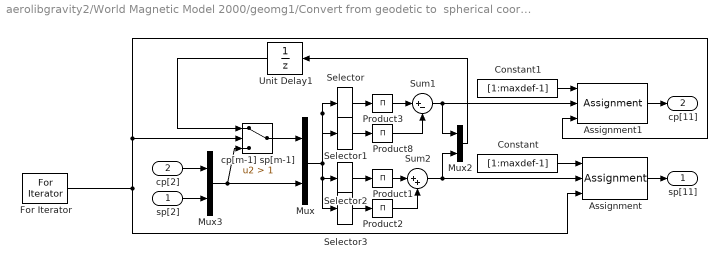
== system aerolibgravity2/World Magnetic Model 2000/geomg1/Convert from geodetic to  spherical coordinates /For Iterator Subsystem ==
  sp[2] : Inport  LatchInput=off
  cp[2] : Inport  Port=2  LatchInput=off
  Assignment : Assignment  ElementSrc=External  DiagnosticForDimensions=Error
  Assignment1 : Assignment  ElementSrc=External  DiagnosticForDimensions=Error
  Constant : Constant  Value=[1:maxdef-1]
  Constant1 : Constant  Value=[1:maxdef-1]
  For Iterator : ForIterator  IterationLimit=maxdef-1  IterationVariableDataType=double
  Mux : Mux  Inputs=[2 2]
  Mux2 : Mux  Inputs=2
  Mux3 : Mux  Inputs=2
  Product{1..3,8} (4 alike) : Product  Inputs=1  SaturateOnIntegerOverflow=on
  Selector : Selector  Elements=[1 3]  InputPortWidth=4
  Selector1 : Selector  Elements=[2 4]  InputPortWidth=4
  Selector2 : Selector  Elements=[1 4]  InputPortWidth=4
  Selector3 : Selector  Elements=[2 3]  InputPortWidth=4
  Sum1 : Sum  Inputs=|+-  SaturateOnIntegerOverflow=on
  Sum2 : Sum  Inputs=|++  SaturateOnIntegerOverflow=on
  Unit Delay1 : UnitDelay  Orientation=left  SampleTime=-1
  cp[m-1] sp[m-1] : Switch  Criteria=u2 > Threshold  Threshold=1  SaturateOnIntegerOverflow=on
  sp[11] : Outport
  cp[11] : Outport  Port=2
  wires:
  Mux3/1 -> cp[m-1] sp[m-1]/3, Mux/2
  Mux2/1 -> Unit Delay1/1
  Selector3/1 -> Product2/1
  Selector2/1 -> Product1/1
  Selector1/1 -> Product8/1
  Mux/1 -> Selector2/1, Selector3/1, Selector1/1, Selector/1
  Selector/1 -> Product3/1
  cp[m-1] sp[m-1]/1 -> Mux/1
  Constant1/1 -> Assignment1/1
  For Iterator/1 -> Assignment/3, cp[m-1] sp[m-1]/2, Assignment1/3
  sp[2]/1 -> Mux3/2
  cp[2]/1 -> Mux3/1
  Assignment1/1 -> cp[11]/1
  Product3/1 -> Sum1/1
  Product8/1 -> Sum1/2
  Product1/1 -> Sum2/1
  Product2/1 -> Sum2/2
  Sum2/1 -> Mux2/2, Assignment/2
  Sum1/1 -> Mux2/1, Assignment1/2
  Unit Delay1/1 -> cp[m-1] sp[m-1]/1
  Assignment/1 -> sp[11]/1
  Constant/1 -> Assignment/1

== system aerolibgravity2/World Magnetic Model 2000/geomg1/Rotate magnetic vector components  to geodetic from spherical and  compute declination, inclination  and total intensity/Calculate bx ==
  ca : Inport  LatchInput=off
  sa : Inport  Port=2  LatchInput=off
  bt : Inport  Port=3  LatchInput=off
  br : Inport  Port=4  LatchInput=off
  Product1 : Product  SaturateOnIntegerOverflow=on
  Product4 : Product  SaturateOnIntegerOverflow=on
  Sum1 : Sum  Inputs=|--  SaturateOnIntegerOverflow=on
  bx : Outport
  wires:
  sa/1 -> Product4/2
  Sum1/1 -> bx/1  "bx"
  ca/1 -> Product1/1
  br/1 -> Product4/1
  bt/1 -> Product1/2
  Product4/1 -> Sum1/2
  Product1/1 -> Sum1/1

== system aerolibgravity2/World Magnetic Model 2000/geomg1/Rotate magnetic vector components  to geodetic from spherical and  compute declination, inclination  and total intensity/Calculate by ==
  bp : Inport  LatchInput=off
  st : Inport  Port=2  LatchInput=off
  bpp : Inport  Port=3  LatchInput=off
  Product : Product  Inputs=*/  SaturateOnIntegerOverflow=on
  Switch : Switch  Criteria=u2 ~= 0  SaturateOnIntegerOverflow=on
  by : Outport
  wires:
  bpp/1 -> Switch/3
  Switch/1 -> by/1  "by"
  bp/1 -> Product/1
  Product/1 -> Switch/1
  st/1 -> Switch/2, Product/2

== system aerolibgravity2/World Magnetic Model 2000/geomg1/Rotate magnetic vector components  to geodetic from spherical and  compute declination, inclination  and total intensity/Calculate bz ==
  ca : Inport  LatchInput=off
  sa : Inport  Port=2  LatchInput=off
  bt : Inport  Port=3  LatchInput=off
  br : Inport  Port=4  LatchInput=off
  Product1 : Product  SaturateOnIntegerOverflow=on
  Product4 : Product  SaturateOnIntegerOverflow=on
  Sum1 : Sum  Inputs=|+-  SaturateOnIntegerOverflow=on
  bz : Outport
  wires:
  Product1/1 -> Sum1/1
  Product4/1 -> Sum1/2
  bt/1 -> Product1/2
  br/1 -> Product4/1
  sa/1 -> Product1/1
  Sum1/1 -> bz/1  "bz"
  ca/1 -> Product4/2

== system aerolibgravity2/World Magnetic Model 2000/geomg1/Rotate magnetic vector components  to geodetic from spherical and  compute declination, inclination  and total intensity/Compute declination, inclination,  and total intensity ==
  by : Inport  LatchInput=off
  bx : Inport  Port=2  LatchInput=off
  bz : Inport  Port=3  LatchInput=off
  Angle Conversion1 : aerolibconvert/Angle Conversion  IU=rad  OU=deg
  Angle Conversion2 : aerolibconvert/Angle Conversion  IU=rad  OU=deg
  Math Function : Math  Operator=sqrt  SaturateOnIntegerOverflow=on
  Math Function1 : Math  Operator=sqrt  SaturateOnIntegerOverflow=on
  Product : Product  SaturateOnIntegerOverflow=on
  Product1 : Product  SaturateOnIntegerOverflow=on
  Product2 : Product  SaturateOnIntegerOverflow=on
  Sum : Sum  Inputs=|++  SaturateOnIntegerOverflow=on
  Sum1 : Sum  Inputs=++|  SaturateOnIntegerOverflow=on
  Trigonometric Function : Trigonometry  Operator=atan2
  Trigonometric Function1 : Trigonometry  Operator=atan2
  dec : Outport
  dip : Outport  Port=2
  ti : Outport  Port=3
  wires:
  Angle Conversion1/1 -> dec/1
  Trigonometric Function1/1 -> Angle Conversion1/1
  Angle Conversion2/1 -> dip/1
  Trigonometric Function/1 -> Angle Conversion2/1
  Math Function1/1 -> Trigonometric Function/2
  Sum1/1 -> Math Function/1
  Product2/1 -> Sum1/1
  Sum/1 -> Sum1/2, Math Function1/1
  Product1/1 -> Sum/2
  Product/1 -> Sum/1
  bz/1 -> Trigonometric Function/1, Product2/2, Product2/1
  bx/1 -> Trigonometric Function1/2, Product1/2, Product1/1
  by/1 -> Trigonometric Function1/1, Product/2, Product/1
  Math Function/1 -> ti/1

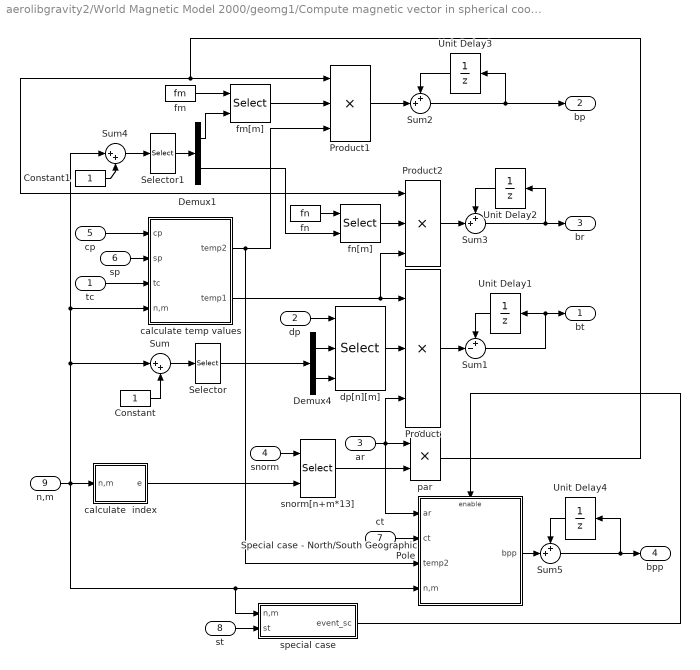
== system aerolibgravity2/World Magnetic Model 2000/geomg1/Compute magnetic vector in spherical coordinates/For Iterator Subsystem/Accumulate terms of the  spherical harmonic expansion ==
  tc : Inport  LatchInput=off
  dp : Inport  Port=2  LatchInput=off
  ar : Inport  Port=3  LatchInput=off
  snorm : Inport  Port=4  LatchInput=off
  cp : Inport  Port=5  LatchInput=off
  sp : Inport  Port=6  LatchInput=off
  ct : Inport  Port=7  LatchInput=off
  st : Inport  Port=8  LatchInput=off
  n,m : Inport  Port=9  LatchInput=off
  Constant : Constant
  Constant1 : Constant
  Demux1 : Demux  Outputs=2
  Demux4 : Demux  Outputs=2
  Product : Product  Inputs=3  SaturateOnIntegerOverflow=on
  Product1 : Product  Inputs=3  SaturateOnIntegerOverflow=on
  Product2 : Product  Inputs=3  SaturateOnIntegerOverflow=on
  Selector : Selector  Elements=[2 1]  InputPortWidth=2
  Selector1 : Selector  Elements=[2 1]  InputPortWidth=2
  Special case - North/South Geographic Pole : Subsystem  TreatAsAtomicUnit=on  PropExecContextAcrossSSBoundary=on
  Sum : Sum  Inputs=|++  SaturateOnIntegerOverflow=on
  Sum1 : Sum  Inputs=+-|  SaturateOnIntegerOverflow=on
  Sum2 : Sum  Inputs=++|  SaturateOnIntegerOverflow=on
  Sum3 : Sum  Inputs=++|  SaturateOnIntegerOverflow=on
  Sum4 : Sum  Inputs=|++  SaturateOnIntegerOverflow=on
  Sum5 : Sum  Inputs=++|  SaturateOnIntegerOverflow=on
  Unit Delay{1..4} (4 alike) : UnitDelay  Orientation=left  SampleTime=-1
  calculate  index : Subsystem  PropExecContextAcrossSSBoundary=on
  calculate temp values : Subsystem  PropExecContextAcrossSSBoundary=on
  dp[n][m] : Selector  InputType=Matrix  ElementSrc=External  Elements=[1 3]  RowSrc=External  ColumnSrc=External  InputPortWidth=maxdef+1
  fm : Constant  Value=fm
  fm[m] : Selector  ElementSrc=External  Elements=[1 3]  InputPortWidth=maxdef+1
  fn : Constant  Value=fn
  fn[m] : Selector  ElementSrc=External  Elements=[1 3]  InputPortWidth=maxdef+1
  par : Product  SaturateOnIntegerOverflow=on
  snorm[n+m*13] : Selector  ElementSrc=External  Elements=[1 3]  InputPortWidth=(maxdef+1)*(maxdef+1)
  special case : Subsystem  PropExecContextAcrossSSBoundary=on
  bt : Outport
  bp : Outport  Port=2
  br : Outport  Port=3
  bpp : Outport  Port=4
  wires:
  special case/1(event_sc) -> Special case - North/South Geographic Pole/Enable
  st/1 -> special case/2(st)
  ct/1 -> Special case - North/South Geographic Pole/2(ct)
  Demux1/2 -> fn[m]/2
  Demux1/1 -> fm[m]/2
  Selector1/1 -> Demux1/1
  Sum4/1 -> Selector1/1
  Constant1/1 -> Sum4/2
  Demux4/2 -> dp[n][m]/3
  Demux4/1 -> dp[n][m]/2
  Selector/1 -> Demux4/1
  Constant/1 -> Sum/2
  Sum/1 -> Selector/1
  tc/1 -> calculate temp values/3(tc)
  Unit Delay2/1 -> Sum3/1
  Sum3/1 -> Unit Delay2/1, br/1
  Product2/1 -> Sum3/2
  fm[m]/1 -> Product1/2
  fn[m]/1 -> Product2/2
  sp/1 -> calculate temp values/2(sp)
  cp/1 -> calculate temp values/1(cp)
  n,m/1 -> special case/1(n,m), Special case - North/South Geographic Pole/4(n,m), Sum4/1, calculate temp values/4(n,m), Sum/1, calculate  index/1(n,m)
  snorm/1 -> snorm[n+m*13]/1
  dp/1 -> dp[n][m]/1
  Unit Delay3/1 -> Sum2/1
  Sum2/1 -> Unit Delay3/1, bp/1
  Product1/1 -> Sum2/2
  fm/1 -> fm[m]/1
  fn/1 -> fn[m]/1
  par/1 -> Product1/1, Product2/1
  calculate temp values/1(temp2) -> Special case - North/South Geographic Pole/3(temp2), Product1/3
  Unit Delay1/1 -> Sum1/1
  Sum1/1 -> Unit Delay1/1, bt/1
  Product/1 -> Sum1/2
  dp[n][m]/1 -> Product/2
  calculate temp values/2(temp1) -> Product/1, Product2/3
  calculate  index/1(e) -> snorm[n+m*13]/2
  ar/1 -> Special case - North/South Geographic Pole/1(ar), par/1, Product/3
  snorm[n+m*13]/1 -> par/2
  Unit Delay4/1 -> Sum5/1
  Sum5/1 -> Unit Delay4/1, bpp/1
  Special case - North/South Geographic Pole/1(bpp) -> Sum5/2

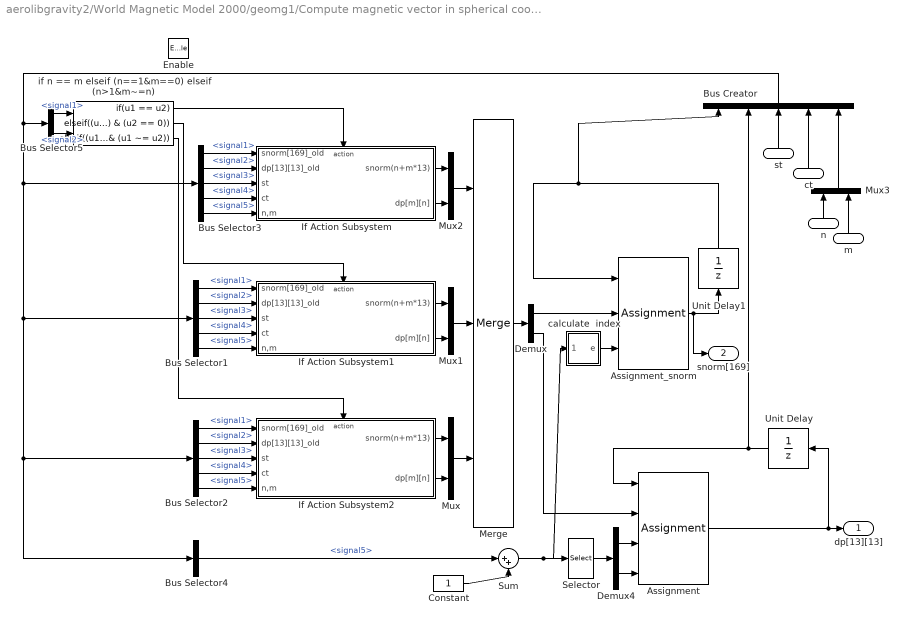
== system aerolibgravity2/World Magnetic Model 2000/geomg1/Compute magnetic vector in spherical coordinates/For Iterator Subsystem/Compute unnormalized associated  legendre polynomials and  derivatives via recursion relations ==
  n : Inport  Orientation=up  LatchInput=off
  m : Inport  Orientation=up  Port=2  LatchInput=off
  st : Inport  Orientation=up  Port=3  LatchInput=off
  ct : Inport  Orientation=up  Port=4  LatchInput=off
  Enable : EnablePort
  Assignment : Assignment  InputType=Matrix  RowSrc=External  ColumnSrc=External  DiagnosticForDimensions=Error
  Assignment_snorm : Assignment  ElementSrc=External  RowSrc=External  ColumnSrc=External  DiagnosticForDimensions=Error
  Bus Creator : BusCreator  Orientation=up  DialogController=Simulink.DDGSource_Bus  Inputs=5
  Bus Selector1 : BusSelector  DialogController=Simulink.DDGSource_Bus  OutputSignals=signal1,signal2,signal3,signal4,signal5
  Bus Selector2 : BusSelector  DialogController=Simulink.DDGSource_Bus  OutputSignals=signal1,signal2,signal3,signal4,signal5
  Bus Selector3 : BusSelector  DialogController=Simulink.DDGSource_Bus  OutputSignals=signal1,signal2,signal3,signal4,signal5
  Bus Selector4 : BusSelector  DialogController=Simulink.DDGSource_Bus  OutputSignals=signal5
  Bus Selector5 : BusSelector  DialogController=Simulink.DDGSource_Bus  OutputSignals=signal5.signal1,signal5.signal2
  Constant : Constant
  Demux : Demux  Outputs=2
  Demux4 : Demux  Outputs=2
  If Action Subsystem : Subsystem  TreatAsAtomicUnit=on  PropExecContextAcrossSSBoundary=on
  If Action Subsystem1 : Subsystem  TreatAsAtomicUnit=on  PropExecContextAcrossSSBoundary=on
  If Action Subsystem2 : Subsystem  TreatAsAtomicUnit=on  PropExecContextAcrossSSBoundary=on
  Merge : Merge  Inputs=3
  Mux : Mux  Inputs=2
  Mux1 : Mux  Inputs=2
  Mux2 : Mux  Inputs=2
  Mux3 : Mux  Orientation=up  Inputs=2
  Selector : Selector  Elements=[2 1]  InputPortWidth=2
  Sum : Sum  Inputs=|++  SaturateOnIntegerOverflow=on
  Unit Delay : UnitDelay  Orientation=left  X0=zeros(maxdef+1,maxdef+1)  SampleTime=-1
  Unit Delay1 : UnitDelay  Orientation=up  X0=snorm  SampleTime=-1
  calculate  index : Subsystem  PropExecContextAcrossSSBoundary=on
  if n == m elseif (n==1&m==0) elseif (n>1&m~=n) : If  NumInputs=2  IfExpression=u1 == u2  ElseIfExpressions=(u1 == 1) & (u2 == 0),(u1 >1) & (u1 ~= u2)  ShowElse=off
  dp[13][13] : Outport
  snorm[169] : Outport  Port=2
  wires:
  Unit Delay1/1 -> Assignment_snorm/1, Bus Creator/1
  Unit Delay/1 -> Bus Creator/2, Assignment/1
  Bus Selector4/1 -> Sum/1  "<signal5>"
  Bus Selector3/5 -> If Action Subsystem/5(n,m)  "<signal5>"
  Bus Selector2/5 -> If Action Subsystem2/5(n,m)  "<signal5>"
  Bus Selector1/5 -> If Action Subsystem1/5(n,m)  "<signal5>"
  m/1 -> Mux3/2
  n/1 -> Mux3/1
  Mux3/1 -> Bus Creator/5
  Selector/1 -> Demux4/1
  Demux4/2 -> Assignment/4
  Demux4/1 -> Assignment/3
  Sum/1 -> Selector/1, calculate  index/1(n,m)
  Bus Selector5/2 -> if n == m elseif (n==1&m==0) elseif (n>1&m~=n)/2  "<signal2>"
  Bus Selector5/1 -> if n == m elseif (n==1&m==0) elseif (n>1&m~=n)/1  "<signal1>"
  Bus Creator/1 -> Bus Selector5/1, Bus Selector3/1, Bus Selector4/1, Bus Selector2/1, Bus Selector1/1
  ct/1 -> Bus Creator/4
  st/1 -> Bus Creator/3
  Bus Selector3/4 -> If Action Subsystem/4(ct)  "<signal4>"
  Bus Selector3/3 -> If Action Subsystem/3(st)  "<signal3>"
  Bus Selector3/2 -> If Action Subsystem/2(dp[13][13]_old)  "<signal2>"
  Bus Selector3/1 -> If Action Subsystem/1(snorm[169]_old)  "<signal1>"
  Bus Selector1/4 -> If Action Subsystem1/4(ct)  "<signal4>"
  Bus Selector1/3 -> If Action Subsystem1/3(st)  "<signal3>"
  Bus Selector1/2 -> If Action Subsystem1/2(dp[13][13]_old)  "<signal2>"
  Bus Selector1/1 -> If Action Subsystem1/1(snorm[169]_old)  "<signal1>"
  Bus Selector2/4 -> If Action Subsystem2/4(ct)  "<signal4>"
  Bus Selector2/3 -> If Action Subsystem2/3(st)  "<signal3>"
  Bus Selector2/2 -> If Action Subsystem2/2(dp[13][13]_old)  "<signal2>"
  Bus Selector2/1 -> If Action Subsystem2/1(snorm[169]_old)  "<signal1>"
  Demux/1 -> Assignment_snorm/2
  Demux/2 -> Assignment/2
  Merge/1 -> Demux/1
  Mux/1 -> Merge/3
  Mux1/1 -> Merge/2
  Mux2/1 -> Merge/1
  If Action Subsystem/2(dp[m][n]) -> Mux2/2
  If Action Subsystem/1(snorm(n+m*13)) -> Mux2/1
  If Action Subsystem1/2(dp[m][n]) -> Mux1/2
  If Action Subsystem1/1(snorm(n+m*13)) -> Mux1/1
  If Action Subsystem2/2(dp[m][n]) -> Mux/2
  If Action Subsystem2/1(snorm(n+m*13)) -> Mux/1
  calculate  index/1(e) -> Assignment_snorm/3
  Assignment_snorm/1 -> snorm[169]/1, Unit Delay1/1
  if n == m elseif (n==1&m==0) elseif (n>1&m~=n)/3 -> If Action Subsystem2/Action
  if n == m elseif (n==1&m==0) elseif (n>1&m~=n)/2 -> If Action Subsystem1/Action
  Assignment/1 -> Unit Delay/1, dp[13][13]/1
  if n == m elseif (n==1&m==0) elseif (n>1&m~=n)/1 -> If Action Subsystem/Action
  Constant/1 -> Sum/2
